simulink model "LUTaeroTest"  (R2025b)
settings: Solver=VariableStepAuto  StartTime=0.0  StopTime=10.0  RelTol=1e-3
libraries: Brown_Flight_Controls_lib x1
settings Model: Creator=zbrown  LastModifiedBy=zbrown

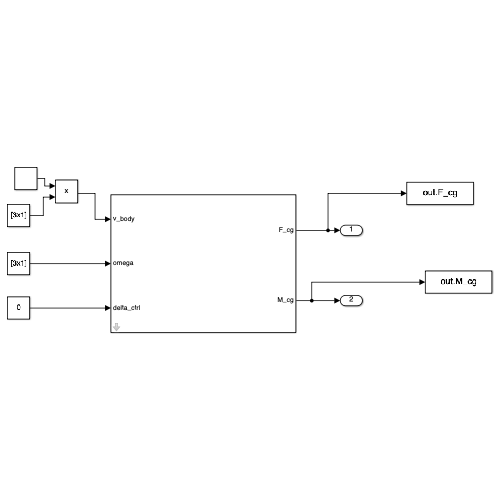
[thumbnail: Simulink's stored preview of the top-level diagram]
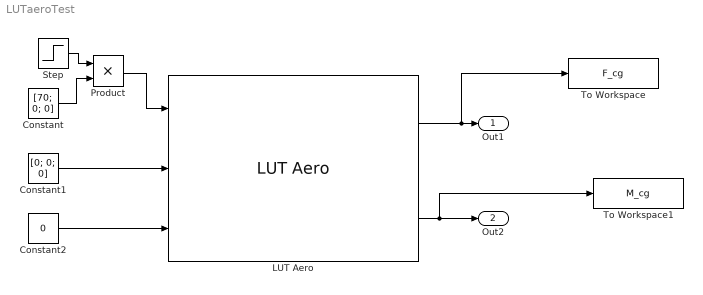
== system LUTaeroTest ==
  Constant : Constant  Value=[70; 0; 0]
  Constant1 : Constant  Value=[0; 0; 0]
  Constant2 : Constant  Value=0
  LUT Aero : Brown_Flight_Controls_lib/LUT Aero  surf=wingR  CG=CG  polar=wingPolar
  Product : Product
  Step : Step  SampleTime=0
  To Workspace : ToWorkspace  VariableName=F_cg  SaveFormat=Timeseries  SampleTime=-1
  To Workspace1 : ToWorkspace  VariableName=M_cg  SaveFormat=Timeseries  SampleTime=-1
  Out1 : Outport
  Out2 : Outport  Port=2
  wires:
  Constant1/1 -> LUT Aero/2
  Constant2/1 -> LUT Aero/3
  LUT Aero/1 -> To Workspace/1, Out1/1
  LUT Aero/2 -> To Workspace1/1, Out2/1
  Step/1 -> Product/1
  Constant/1 -> Product/2
  Product/1 -> LUT Aero/1
